simulink model "SimHinfLong2020b"  (R2021b)
settings: Solver=VariableStepAuto  StartTime=0.0  StopTime=15  RelTol=1e-3
values from neighbouring files (symbols this model uses):
  Along = [-0.596109126676 -0.745393804819 1.04174439924 0 -0.0537687381563 135.84300719 0.801088301065 -7.58095179424 -7.4269344992 0 0.998551936758 7.31469923109 ... (36 elements, 6x6)]    [modelo_lin.mat]
  Blong = [-0.596109126676 -0.745393804819 1.04174439924 0 -0.0537687381563 135.84300719 0.801088301065 -7.58095179424 -7.4269344992 0 0.998551936758 7.31469923109 ... (36 elements, 6x6)]    [modelo_lin.mat]
  Clong = [-0.596109126676 -0.745393804819 1.04174439924 0 -0.0537687381563 135.84300719 0.801088301065 -7.58095179424 -7.4269344992 0 0.998551936758 7.31469923109 ... (36 elements, 6x6)]    [modelo_lin.mat]
  Dlong = [-0.596109126676 -0.745393804819 1.04174439924 0 -0.0537687381563 135.84300719 0.801088301065 -7.58095179424 -7.4269344992 0 0.998551936758 7.31469923109 ... (36 elements, 6x6)]    [modelo_lin.mat]
undefined symbols (not defined in the file or in its folder): K
libraries: simulink x1
settings Model: Creator=danie  LastModifiedBy=Daniel
settings SolverCC: AlgebraicLoopSolver=TrustRegion
settings DebuggingCC: UnconnectedInputMsg=none  UnconnectedOutputMsg=none  UnconnectedLineMsg=none

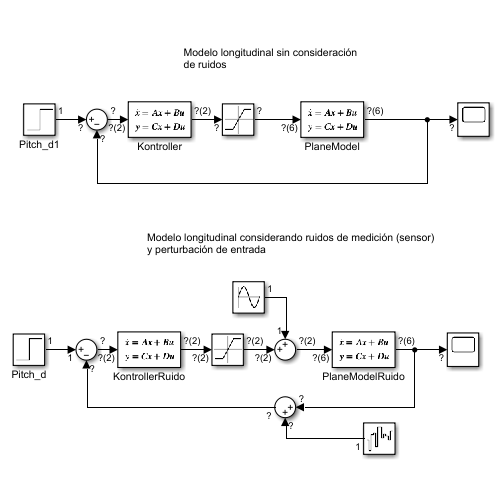
[thumbnail: Simulink's stored preview of the top-level diagram]
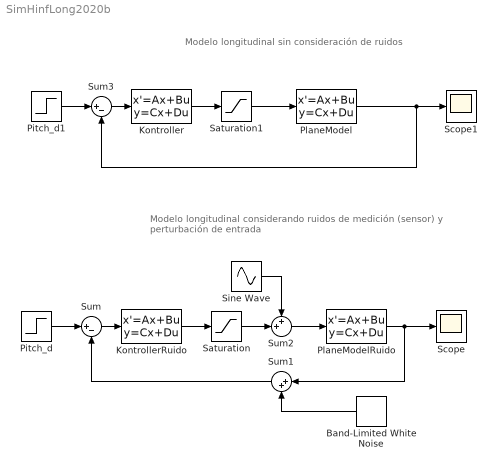
== system SimHinfLong2020b ==
  note: Modelo longitudinal sin consideración
      | de ruidos
  note: Modelo longitudinal considerando ruidos de medición (sensor)
      | y perturbación de entrada
  Band-Limited White Noise : simulink/Sources/Band-Limited White Noise  Cov=[0.0001]  Ts=0.1  seed=[23341]
  Kontroller : StateSpace  A=K.A  B=K.B  C=K.C  D=K.D  InitialCondition=0
  KontrollerRuido : StateSpace  A=K.A  B=K.B  C=K.C  D=K.D  InitialCondition=0
  Pitch_d : Step  After=40  SampleTime=0
  Pitch_d1 : Step  After=40  SampleTime=0
  PlaneModel : StateSpace  A=Along  B=Blong  C=Clong  D=Dlong  InitialCondition=0
  PlaneModelRuido : StateSpace  A=Along  B=Blong  C=Clong  D=Dlong  InitialCondition=0
  Saturation : Saturate  UpperLimit=30  LowerLimit=-30
  Saturation1 : Saturate  UpperLimit=30  LowerLimit=-30
  Scope : Scope
  Scope1 : Scope
  Sine Wave : Sin  Frequency=12*pi  SampleTime=0
  Sum : Sum  Inputs=|+-
  Sum1 : Sum  Inputs=|++
  Sum2 : Sum  Inputs=++|
  Sum3 : Sum  Inputs=|+-
  wires:
  KontrollerRuido/1 -> Saturation/1
  Sum/1 -> KontrollerRuido/1
  Pitch_d/1 -> Sum/1
  PlaneModelRuido/1 -> Sum1/1, Scope/1
  Band-Limited White Noise/1 -> Sum1/2
  Sum1/1 -> Sum/2
  Saturation/1 -> Sum2/2
  Sum2/1 -> PlaneModelRuido/1
  Sine Wave/1 -> Sum2/1
  Saturation1/1 -> PlaneModel/1
  PlaneModel/1 -> Sum3/2, Scope1/1
  Pitch_d1/1 -> Sum3/1
  Kontroller/1 -> Saturation1/1
  Sum3/1 -> Kontroller/1
